simulink model "SimpleHeatexchanger_std"  (R2023b)
settings: Solver=ode4  StartTime=0.0  StopTime=10.0  FixedStep=1e-4  RelTol=1e-6
undefined symbols (not defined in the file): p_in, RH_in, T_in, W_in, yO2_in
libraries: slpidlib x1
settings Model: Creator=KOTA-Z  LastModifiedBy=KOTA-Z

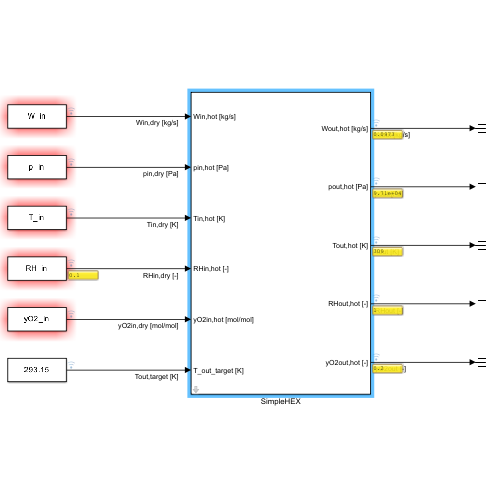
[thumbnail: Simulink's stored preview of the top-level diagram]
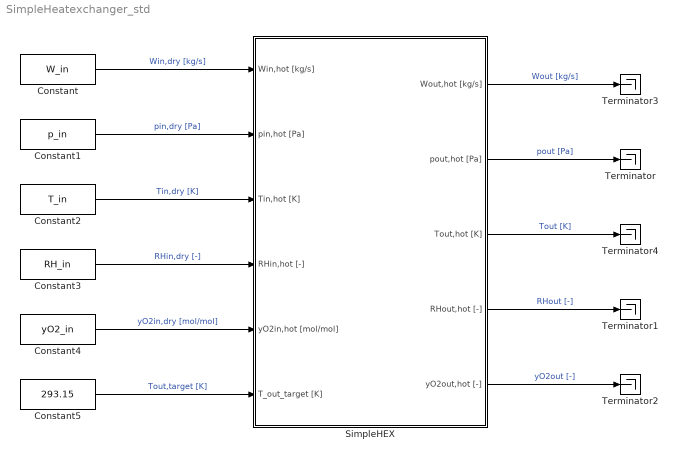
== system SimpleHeatexchanger_std ==
  Constant : Constant  Value=W_in
  Constant1 : Constant  Value=p_in
  Constant2 : Constant  Value=T_in
  Constant3 : Constant  Value=RH_in
  Constant4 : Constant  Value=yO2_in
  Constant5 : Constant  Value=293.15
  SimpleHEX : Subsystem  mask(Simple FCstack){eta_hex=0.8, T_cool=293.15, cp_cool=4185}
      mask prompts: eta_hex "Efficiency of HEX [-]"; T_cool "Temperature of coolant [K]"; cp_cool "cp of coolant [J/kg/K]"
      mask help: This block provides a simplified FCstack model. The reacted O2 and generated H2O in the stack are calculated based on lambda. Delay due to volume is considered and the pressure drop is approximated as the orifice law.
      mask DialogControl Container3 Prompt: Heatexchanger Parameter
  Terminator{,1..4} (5 alike) : Terminator
  wires:
  Constant4/1 -> SimpleHEX/5(yO2in,hot [mol/mol])  "yO2in,dry [mol/mol]"
  Constant/1 -> SimpleHEX/1(Win,hot [kg/s])  "Win,dry [kg/s]"
  Constant3/1 -> SimpleHEX/4(RHin,hot [-])  "RHin,dry [-]"
  Constant1/1 -> SimpleHEX/2(pin,hot [Pa])  "pin,dry [Pa]"
  SimpleHEX/4(RHout,hot [-]) -> Terminator1/1  "RHout [-]"
  SimpleHEX/1(Wout,hot [kg/s]) -> Terminator3/1  "Wout [kg/s]"
  SimpleHEX/2(pout,hot [Pa]) -> Terminator/1  "pout [Pa]"
  SimpleHEX/5(yO2out,hot [-]) -> Terminator2/1  "yO2out [-]"
  Constant2/1 -> SimpleHEX/3(Tin,hot [K])  "Tin,dry [K]"
  SimpleHEX/3(Tout,hot [K]) -> Terminator4/1  "Tout [K]"
  Constant5/1 -> SimpleHEX/6(T_out_target [K])  "Tout,target [K]"

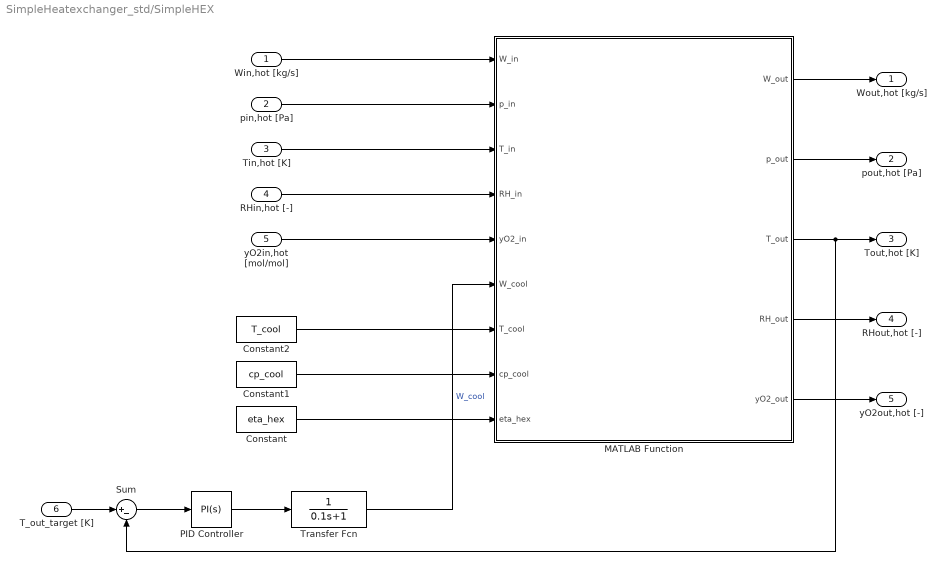
== system SimpleHeatexchanger_std/SimpleHEX ==
  Win,hot [kg/s] : Inport
  pin,hot [Pa] : Inport  Port=2
  Tin,hot [K] : Inport  Port=3
  RHin,hot [-] : Inport  Port=4
  yO2in,hot [mol/mol] : Inport  Port=5
  T_out_target [K] : Inport  Port=6
  Constant : Constant  Value=eta_hex
  Constant1 : Constant  Value=cp_cool
  Constant2 : Constant  Value=T_cool
  MATLAB Function : MATLAB Function  TreatAsAtomicUnit=on
  PID Controller : slpidlib/PID Controller  Controller=PI  Form=Parallel  TimeDomain=Continuous-time  UseExternalTs=off  SampleTime=-1  IntegratorMethod=Forward Euler  FilterMethod=Forward Euler  ControllerParametersSource=internal  P=-0.01  I=-0.1  UseKiTs=off  D=0  N=100  UseFilter=on  TunerSelectOption=Transfer Function Based (PID Tuner App)  InitialConditionSource=internal  InitialConditionForIntegrator=0  InitialConditionForFilter=0  DifferentiatorICPrevScaledInput=0  ExternalReset=none  TrackingMode=off  Kt=1  LimitOutput=on  SatLimitsSource=internal  UpperSaturationLimit=2  LowerSaturationLimit=0  LinearizeAsGain=on  AntiWindupMode=back-calculation  Kb=1  LimitIntegrator=off  UpperIntegratorSaturationLimit=inf  LowerIntegratorSaturationLimit=-inf  POutMin=[]  POutMax=[]  IOutMin=[]  IOutMax=[]  DOutMin=[]  DOutMax=[]  NOutMin=[]  NOutMax=[]  SumOutMin=[]  SumOutMax=[]  SaturationOutMin=[]  SaturationOutMax=[]  PParamMin=[]  PParamMax=[]  IParamMin=[]  IParamMax=[]  DParamMin=[]  DParamMax=[]  NParamMin=[]  NParamMax=[]  KbParamMin=[]  KbParamMax=[]  KtParamMin=[]  KtParamMax=[]  KbOutMin=[]  KbOutMax=[]  KtOutMin=[]  KtOutMax=[]  IntegratorOutMin=[]  IntegratorOutMax=[]  FilterOutMin=[]  FilterOutMax=[]  SumI1OutMin=[]  SumI1OutMax=[]  SumI2OutMin=[]  SumI2OutMax=[]  SumI3OutMin=[]  SumI3OutMax=[]  SumI4OutMin=[]  SumI4OutMax=[]  SumDOutMin=[]  SumDOutMax=[]  DifferentiatorOutMin=[]  DifferentiatorOutMax=[]  FilterDiffOutCoefMin=[]  FilterDiffOutCoefMax=[]  ReciprocalOutMin=[]  ReciprocalOutMax=[]  SumDenOutMin=[]  SumDenOutMax=[]  SumNumOutMin=[]  SumNumOutMax=[]  DivideOutMin=[]  DivideOutMax=[]  UdiffTsProdOutMin=[]  UdiffTsProdOutMax=[]  NTsProdOutMin=[]  NTsProdOutMax=[]  UintegralTsProdOutMin=[]  UintegralTsProdOutMax=[]  UngainTsProdOutMin=[]  UngainTsProdOutMax=[]  ClampingZeroOutDataTypeStr=Inherit: Inherit via back propagation  ClampingZeroOutMin=[]  ClampingZeroOutMax=[]  FilterDenConstantOutDataTypeStr=Inherit: Inherit via back propagation  FilterDenConstantOutMin=[]  FilterDenConstantOutMax=[]  PCopyOutDataTypeStr=Inherit: Inherit via back propagation  PCopyOutMin=[]  PCopyOutMax=[]  NCopyOutDataTypeStr=Inherit: Inherit via back propagation  NCopyOutMin=[]  NCopyOutMax=[]  IntegratorContinuousStateAttributes=''  IntegratorStateMustResolveToSignalObject=off  IntegratorRTWStateStorageClass=Auto  FilterContinuousStateAttributes=''  FilterStateMustResolveToSignalObject=off  FilterRTWStateStorageClass=Auto  ParallelPVariant=InternalParameters  IdealPVariant=Disabled  IVariant=InternalParameters  DVariant=Disabled  IntegratorVariant=Continuous  SatVariant=Enabled  AWVariant=BackCalculation  PCopyVariant=Disabled  TRVariant=Disabled  FdbkBlocksVariant=Forward  IdealPFdbkVariant=Disabled  SatFdbkVariant=Disabled  DerivativeFilterVariant=Disabled  NVariant=Disabled  NCopyVariant=Disabled_SignalSpec  FilterICVariant=Disabled  IntegratorICVariant=InternalICs  ExternalResetVariant=Disabled  TRSumVariant=Passthrough  SumFdbkVariant=Disabled  SumVariant=Sum_PI  TsampFilterVariant=InternalTs  TsampNgainVariant=Passthrough  TsampIntegralVariant=Disabled_SignalSpec  ExternalSaturationOutDataTypeStr=Inherit: Same as second input
  Sum : Sum  Inputs=|+-
  Transfer Fcn : TransferFcn  Denominator=[0.1 1]
  Wout,hot [kg/s] : Outport
  pout,hot [Pa] : Outport  Port=2
  Tout,hot [K] : Outport  Port=3
  RHout,hot [-] : Outport  Port=4
  yO2out,hot [-] : Outport  Port=5
  wires:
  MATLAB Function/5(yO2_out) -> yO2out,hot [-]/1
  MATLAB Function/2(p_out) -> pout,hot [Pa]/1
  MATLAB Function/1(W_out) -> Wout,hot [kg/s]/1
  MATLAB Function/4(RH_out) -> RHout,hot [-]/1
  MATLAB Function/3(T_out) -> Sum/2, Tout,hot [K]/1
  RHin,hot [-]/1 -> MATLAB Function/4(RH_in)
  pin,hot [Pa]/1 -> MATLAB Function/2(p_in)
  Tin,hot [K]/1 -> MATLAB Function/3(T_in)
  Win,hot [kg/s]/1 -> MATLAB Function/1(W_in)
  yO2in,hot [mol/mol]/1 -> MATLAB Function/5(yO2_in)
  PID Controller/1 -> Transfer Fcn/1
  Transfer Fcn/1 -> MATLAB Function/6(W_cool)  "W_cool"
  Sum/1 -> PID Controller/1
  T_out_target [K]/1 -> Sum/1
  Constant2/1 -> MATLAB Function/7(T_cool)
  Constant1/1 -> MATLAB Function/8(cp_cool)
  Constant/1 -> MATLAB Function/9(eta_hex)

== matlab function SimpleHeatexchanger_std/SimpleHEX/MATLAB Function ==
  data: W_in input; W_out output; p_in input; T_in input; RH_in input; yO2_in input; W_cool input; p_out output; T_out output; RH_out output; yO2_out output; T_cool input; cp_cool input; eta_hex input
%% 伝熱計算
function [W_out, p_out, T_out, RH_out, yO2_out] = HEX_std(W_in, p_in, T_in, RH_in, yO2_in, W_cool, T_cool, cp_cool, eta_hex)
    % 湿り空気の状態計算
    [W_O2_in, W_N2_in, W_vp_in, p_O2_in, p_N2_in, p_vp_in, M_in, R_in, cp_in, kap_in] = calc_MA_property(W_in, p_in, T_in, RH_in, yO2_in);

    % 熱容量の計算
    C_hot  = cp_in * W_in;
    C_cold = cp_cool * W_cool;
    C_min = min(C_hot,C_cold);
    % 熱交換量計算
    Q_hex = eta_hex * C_min*(T_in - T_cool);

    % 出口温度の計算
    if W_in <= 0
        T_out = T_in;
    else
        T_out = T_in - Q_hex/(cp_in*W_in);
    end

    % 相対湿度計算
    RH_out = p_vp_in/sat_vp_pressure(T_out);
    if RH_out < 1
        % 流量は一定とする
        W_out = W_in;       % [kg/s]
        % 圧力は一定とする
        p_out = p_in;       % [Pa]
    else
        RH_out = 1;
        % 凝縮した分の減圧量を加味
        p_vp_out = sat_vp_pressure(T_out);
        p_out = p_O2_in + p_N2_in + p_vp_out;
        % 凝縮した分の流量減少を加味
        p_vp_out = sat_vp_pressure(T_out);
        if p_vp_in <= 0
            W_vp_out = 0;
        else
            W_vp_out = p_vp_out/p_vp_in * W_vp_in;
        end
        W_out = W_O2_in + W_N2_in + W_vp_out;

    end

    % 空気組成は一定とする
    yO2_out = yO2_in;   % [-]
end


%% 湿り空気の状態量計算
function [W_O2, W_N2, W_vp, p_O2, p_N2, p_vp, M, R, cp, kap] = calc_MA_property(W, p, T, RH, yO2)
    % 物理定数の定義
    % 分子量定義
    M_O2 = 32e-3;   % [kg/mol]
    M_N2 = 28e-3;   % [kg/mol]
    M_vp = 18e-3;   % [kg/mol]
    % 気体定数定義
    R0 = 8.31446261815324; % [J/K/mol]
    
    % 分圧計算
    p_vp_sat = sat_vp_pressure(T);
    p_vp = RH * p_vp_sat;
    p_DA = p - p_vp;
    p_O2 = yO2 * p_DA;
    p_N2 = p_DA - p_O2;
    
    % 湿り空気のモル分率計算
    x_O2 = p_O2/p;
    x_N2 = p_N2/p;
    x_vp = p_vp/p;

    % 湿り空気の分子量計算
    M = M_O2*x_O2 + M_N2*x_N2 + M_vp*x_vp;       % [kg/mol]

    % ガス定数計算
    R = R0/M;   % [J/K/kg]

    % 質量分率計算
    w_O2 = x_O2*M_O2 / M;
    w_N2 = x_N2*M_N2 / M;
    w_vp = x_vp*M_vp / M;

    % 各分子の定圧比熱の計算
    % 二原子分子
    cp_O2 = 7/2*R0 / M_O2;  % [J/K/kg]
    cp_N2 = 7/2*R0 / M_N2;  % [J/K/kg]
    % 水蒸気
    cp_vp = 4*R0 / M_vp;    % [J/K/kg]

    % 混合気体の定圧比熱
    cp = cp_O2*w_O2 + cp_N2*w_N2 + cp_vp*w_vp;  % [J/K/kg]

    % 混合気体の比熱比
    kap = cp/(cp-R);

    % 各分子の質量流量
    W_O2 = W * w_O2;    % [kg/s]
    W_N2 = W * w_N2;    % [kg/s]
    W_vp = W * w_vp;    % [kg/s]
end

%% Calculate saturated vapor pressure [Pa]
function psat = sat_vp_pressure(Ts)
    P_CONVERT = 0.001;
    C1 = -5.6745359e3;
    C2 = 6.3925247;
    C3 = -9.6778430e-3;
    C4 = 6.2215701e-7;
    C5 = 2.0747825e-9;
    C6 = -9.4840240e-13;
    C7 = 4.1635019;
    N1 = 0.11670521452767e4;
    N2 = -0.72421316703206e6;
    N3 = -0.17073846940092e2;
    N4 = 0.12020824702470e5;
    N5 = -0.32325550322333e7;
    N6 = 0.14915108613530e2;
    N7 = -0.4823265731591e4;
    N8 = 0.40511340542057e6;
    N9 = -0.23855557567849e0;
    N10 = 0.65017534844798e3;
    
    if Ts < 273.15+0.01
        % -100~0.01C//三重点を計算以下は wexler-hyland のシミュレーションプログラム式
        psat = exp(C1 / Ts + C2 + C3 * Ts + C4 * Ts^2 + C5 * Ts^3 + C6 * Ts^4 + C7 * log(Ts)) * P_CONVERT;
    else
        %　~647.096K//臨界温度まで一定とするは IAPWS-IF97 実用国際状態式
        alpha = Ts + N9 / (Ts - N10);
        a2 = alpha * alpha;
        A = a2 + N1 * alpha + N2;
        B = N3 * a2 + N4 * alpha + N5;
        C = N6 * a2 + N7 * alpha + N8;
        psat = (2 * C / (-B + (B * B - 4 * A * C)^0.5))^4 / P_CONVERT;
    end 
    psat = psat*1000; %kPa to Pa
end
